simulink model "atrias_on_boom"  (R2018b)
settings: Solver=ode15s  StartTime=0.0  StopTime=inf  FixedStep=sample_time  MaxStep=1e-2  RelTol=1e-3
InitFcn:
  | addpath('../common/')
  | colors
  | simulation_params
  | mechanical_params
StartFcn:
  | clc
  | tic
StopFcn:
  | stopscript
values from neighbouring files (symbols this model uses):
  sample_time = 1/sample_freq    (= 0.001)    [simulation_params.m]
undefined symbols (not defined in the file or in its folder): Force_Control, rad, s, sgn, sm, t_friction, X, Y, Z
libraries: sm_lib x205, nesl_utility x123, simulink x49, fl_lib x16, mblibv1 x4, simulink_extras x2, powerlib_meascontrol x1
(part 5 of 8)

== system atrias_on_boom/Mechanical System Layer/R Leg/Thigh SEA ==
  note: Thigh SEA Mechanics
  Thigh Gear Torque [Nm] : Inport
  Thigh Joint [rad rad/s] : Inport  Port=2
  Continuous Angle : mblibv1/Utilities/Continuous Angle  rad=rad  rads=rad/s
      settings: SourceProductName=Simscape  SourceProductBaseCode=SS
  Demux : Demux  Outputs=2
  Gain : Gain  Gain=sm.k_leg_spring
  Gain1 : Gain  Gain=sm.b_leg_spring
  Initial Gear Angle : Constant  Value=sm.thigh_initial_r
  Inverse Gear Ratio1 : Gain  Gain=1/sm.N
  Inverse Gear Ratio2 : Gain  Gain=sm.Kt_leg
  Inverse Gear Ratio3 : Gain  Gain=1/sm.Kt_leg
  Motor Direction : Gain  Gain=-1
  Motor Efficiency : Gain  Gain=sm.mu_motor
  Motor Controller : Subsystem  Commented=on
  Motor Electromagnetism : Subsystem  Commented=on
  Rotor Damping : Gain  Gain=sm.b_rotor
  Rotor and Gearing : Subsystem
  Sum : Sum  Inputs=++|
  Sum2 : Sum  Inputs=+|-
  Sum3 : Sum  Inputs=|+-
  Sum4 : Sum  Inputs=+|-
  Sum5 : Sum  Inputs=|++
  Torque Limiter (outside) 2 : Saturate  UpperLimit=sm.LEG_MTR_MAX_TORQUE  LowerLimit=-sm.LEG_MTR_MAX_TORQUE  ZeroCross=off
      settings: AttributesFormatString=Hi: %<UpperLimit>\nLo: %<LowerLimit>
  Rotor Joint Conn : PMIOPort  Side=Left
  Thigh Joint Torque [Nm] : Outport
  Thigh Gear [rad] : Outport  Port=2
  wires:
  Sum2/1 -> Gain/1
  Sum3/1 -> Motor Efficiency/1
  Rotor Damping/1 -> Sum3/2
  Gain/1 -> Sum5/1  "tau_load"
  Gain1/1 -> Sum5/2
  Sum4/1 -> Gain1/1
  Thigh Joint [rad rad/s]/1 -> Demux/1
  Demux/1 -> Sum2/2
  Demux/2 -> Sum4/2
  Inverse Gear Ratio3/1 -> Inverse Gear Ratio2/1
  Inverse Gear Ratio2/1 -> Sum3/1
  Initial Gear Angle/1 -> Sum/1
  Sum/1 -> Thigh Gear [rad]/1, Sum2/1
  Continuous Angle/1 -> Sum/2
  Rotor and Gearing/1(Gearhead Position [rad]) -> Continuous Angle/1
  Motor Controller/1(Voltage [V]) -> Motor Electromagnetism/1(Voltage [V])
  Motor Electromagnetism/1(Current [A]) -> Motor Controller/2(Measured Current [A])
  Thigh Gear Torque [Nm]/1 -> Motor Direction/1
  Inverse Gear Ratio1/1 -> Inverse Gear Ratio3/1
  Motor Efficiency/1 -> Rotor and Gearing/1(Rotor Torque [Nm])
  Rotor and Gearing/2(Gearhead Velocity [rad/s]) -> Sum4/1, Continuous Angle/2
  Sum5/1 -> Thigh Joint Torque [Nm]/1, Rotor and Gearing/2(Spring Torque [Nm])
  Rotor and Gearing/3(Rotor Velocity [rad/s]) -> Rotor Damping/1
  Torque Limiter (outside) 2/1 -> Inverse Gear Ratio1/1
  Motor Direction/1 -> Torque Limiter (outside) 2/1
  connections:
  Rotor and Gearing/LConn1 -- Rotor Joint Conn/RConn1

== system atrias_on_boom/Mechanical System Layer/Right Hip Roll Joint/Mechanical Limits  ==
  vphi : Inport
  phi : Inport  Port=2
  Compare To Constant5 : simulink/Logic and Bit Operations/Compare To Constant  relop=<=  const=sm.phi_max_collision  OutDataTypeStr=boolean  ZeroCross=off
  Compare To Zero1 : simulink/Logic and Bit Operations/Compare To Zero  relop=<=  OutDataTypeStr=boolean  ZeroCross=off
  Compare To Zero2 : simulink/Logic and Bit Operations/Compare To Zero  relop=<=  OutDataTypeStr=boolean  ZeroCross=off
  Constant1 : Constant  Value=sm.phi_roll_min
  Constant2 : Constant  Value=sm.phi_roll_max
  Enabled Subsystem : Subsystem  TreatAsAtomicUnit=on
  Gain2 : Gain  Gain=-1
  Logical Operator : Logic  Operator=OR  Inputs=1  AllPortsSameDT=off  OutDataTypeStr=boolean
  Mux : Mux  Inputs=2
  Roll Max Collision Model : Subsystem
  Roll Min Collision Model : Subsystem
  Stop Simulation6 : Stop
  Sum1 : Sum  Inputs=-+|
  Sum11 : Sum  Inputs=-|+
  Sum5 : Sum  Inputs=+-|
  tau_reaction : Outport
  wires:
  Sum1/1 -> [col_hip_min], Compare To Zero1/1, Roll Min Collision Model/1(phi [rad])
  Roll Min Collision Model/1(tau_interaction[Nm]) -> Sum11/2
  Compare To Zero1/1 -> Roll Min Collision Model/Enable
  phi/1 -> Sum1/2, Sum5/2
  Logical Operator/1 -> Stop Simulation6/1, Enabled Subsystem/Enable
  [col_hip_max] -> Mux/1
  Mux/1 -> Compare To Constant5/1
  [col_hip_min] -> Mux/2
  Sum11/1 -> tau_reaction/1
  Constant1/1 -> Sum1/1
  Compare To Constant5/1 -> Enabled Subsystem/1(Col_Flags), Logical Operator/1
  Constant2/1 -> Sum5/1
  Sum5/1 -> [col_hip_max], Compare To Zero2/1, Roll Max Collision Model/1(phi [rad])
  Compare To Zero2/1 -> Roll Max Collision Model/Enable
  Roll Max Collision Model/1(tau_interaction[Nm]) -> Sum11/1
  vphi/1 -> Roll Min Collision Model/2(vphi [rad/s]), Gain2/1
  Gain2/1 -> Roll Max Collision Model/2(vphi [rad/s])

== system atrias_on_boom/Mechanical System Layer/Torso/Frame Data ==
  Kinematic Data : ToWorkspace  VariableName=torso_out  SampleTime=sm.output_sample_time
      settings: Save2DSignal=2-D array (concatenate along first dimension)
  Mux : Mux
  PS-Simulink Converter{,1..3} (4 alike) : nesl_utility/PS-Simulink Converter  PhysicalDomain=network_engine_domain  SubClassName=ps_output  LeftPortType=input  RightPortType=output  PseudoPeriodic=off  Frequencies=[]  Unit=1  AffineConversion=off
  Transform Sensor : sm_lib/Frames and Transforms/Transform Sensor  MeasurementFrame=World  SenseAngle=off  SenseAxis=off  SenseAngle1=off  SenseAngle2=off  SenseAngle3=off  SenseQ=on  SenseR=off  SenseOmegaX=off  SenseOmegaY=off  SenseOmegaZ=off  SenseOmega1=off  SenseOmega2=off  SenseOmega3=off  SenseQDot=off  SenseRDot=off  SenseAlphaX=off  SenseAlphaY=off  SenseAlphaZ=off  SenseAlpha1=off  SenseAlpha2=off  SenseAlpha3=off  SenseQDDot=off  SenseRDDot=off  SenseX=on  SenseY=on  SenseZ=on  SenseRad=off  SenseAzim=off  SenseDist=off  SenseInc=off  SenseXDot=off  SenseYDot=off  SenseZDot=off  SenseRadDot=off  SenseAzimDot=off  SenseDistDot=off  SenseIncDot=off  SenseXDDot=off  SenseYDDot=off  SenseZDDot=off  SenseRadDDot=off  SenseAzimDDot=off  SenseDistDDot=off  SenseIncDDot=off
  World Frame : sm_lib/Frames and Transforms/World Frame
  Frame : PMIOPort  Side=Left
  wires:
  Mux/1 -> Kinematic Data/1
  PS-Simulink Converter/1 -> Mux/1
  PS-Simulink Converter1/1 -> Mux/2
  PS-Simulink Converter2/1 -> Mux/3
  PS-Simulink Converter3/1 -> Mux/4
  connections:
  PS-Simulink Converter3/LConn1 -- Transform Sensor/RConn5
  PS-Simulink Converter2/LConn1 -- Transform Sensor/RConn4
  PS-Simulink Converter1/LConn1 -- Transform Sensor/RConn3
  PS-Simulink Converter/LConn1 -- Transform Sensor/RConn2
  Transform Sensor/RConn1 -- Frame/RConn1
  Transform Sensor/LConn1 -- World Frame/RConn1

== system atrias_on_boom/Mechanical System Layer/Yaw Shaft/Frame Data ==
  Kinematic Data : ToWorkspace  VariableName=boom_yaw_out  SampleTime=sm.output_sample_time
      settings: Save2DSignal=2-D array (concatenate along first dimension)
  Mux : Mux
  PS-Simulink Converter{,1..3} (4 alike) : nesl_utility/PS-Simulink Converter  PhysicalDomain=network_engine_domain  SubClassName=ps_output  LeftPortType=input  RightPortType=output  PseudoPeriodic=off  Frequencies=[]  Unit=1  AffineConversion=off
  Transform Sensor : sm_lib/Frames and Transforms/Transform Sensor  MeasurementFrame=World  SenseAngle=off  SenseAxis=off  SenseAngle1=off  SenseAngle2=off  SenseAngle3=off  SenseQ=on  SenseR=off  SenseOmegaX=off  SenseOmegaY=off  SenseOmegaZ=off  SenseOmega1=off  SenseOmega2=off  SenseOmega3=off  SenseQDot=off  SenseRDot=off  SenseAlphaX=off  SenseAlphaY=off  SenseAlphaZ=off  SenseAlpha1=off  SenseAlpha2=off  SenseAlpha3=off  SenseQDDot=off  SenseRDDot=off  SenseX=on  SenseY=on  SenseZ=on  SenseRad=off  SenseAzim=off  SenseDist=off  SenseInc=off  SenseXDot=off  SenseYDot=off  SenseZDot=off  SenseRadDot=off  SenseAzimDot=off  SenseDistDot=off  SenseIncDot=off  SenseXDDot=off  SenseYDDot=off  SenseZDDot=off  SenseRadDDot=off  SenseAzimDDot=off  SenseDistDDot=off  SenseIncDDot=off
  World Frame : sm_lib/Frames and Transforms/World Frame
  Frame : PMIOPort  Side=Left
  wires:
  Mux/1 -> Kinematic Data/1
  PS-Simulink Converter/1 -> Mux/1
  PS-Simulink Converter1/1 -> Mux/2
  PS-Simulink Converter2/1 -> Mux/3
  PS-Simulink Converter3/1 -> Mux/4
  connections:
  PS-Simulink Converter3/LConn1 -- Transform Sensor/RConn5
  PS-Simulink Converter2/LConn1 -- Transform Sensor/RConn4
  PS-Simulink Converter1/LConn1 -- Transform Sensor/RConn3
  PS-Simulink Converter/LConn1 -- Transform Sensor/RConn2
  Transform Sensor/RConn1 -- Frame/RConn1
  Transform Sensor/LConn1 -- World Frame/RConn1

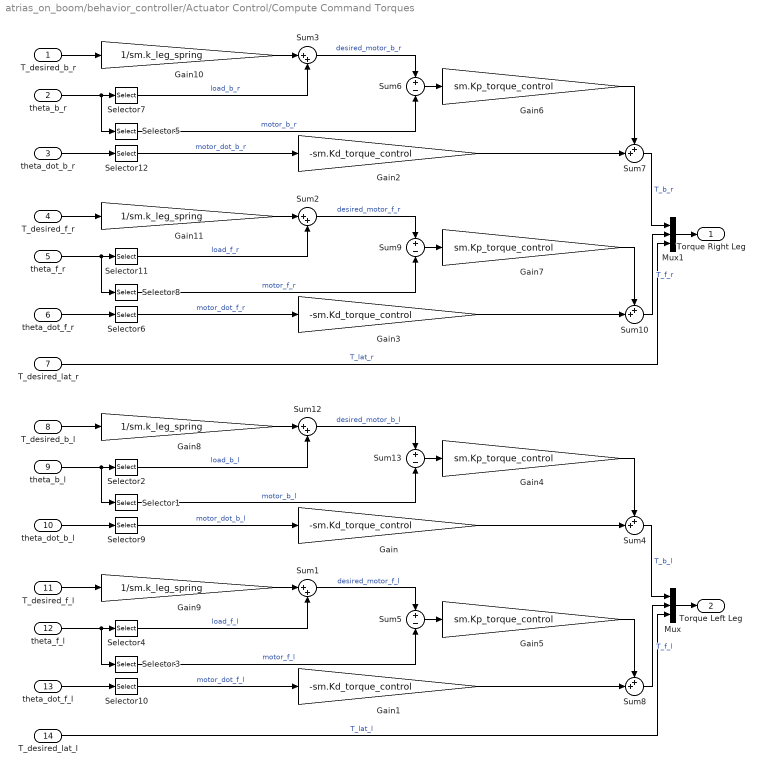
== system atrias_on_boom/behavior_controller/Actuator Control/Compute Command Torques ==
  T_desired_b_r : Inport
  theta_b_r : Inport  Port=2
  theta_dot_b_r : Inport  Port=3
  T_desired_f_r : Inport  Port=4
  theta_f_r : Inport  Port=5
  theta_dot_f_r : Inport  Port=6
  T_desired_lat_r : Inport  Port=7
  T_desired_b_l : Inport  Port=8
  theta_b_l : Inport  Port=9
  theta_dot_b_l : Inport  Port=10
  T_desired_f_l : Inport  Port=11
  theta_f_l : Inport  Port=12
  theta_dot_f_l : Inport  Port=13
  T_desired_lat_l : Inport  Port=14
  Gain{,1..3} (4 alike) : Gain  Gain=-sm.Kd_torque_control
  Gain{8..11} (4 alike) : Gain  Gain=1/sm.k_leg_spring
  Gain{4..7} (4 alike) : Gain  Gain=sm.Kp_torque_control
  Mux : Mux  Inputs=3
  Mux1 : Mux  Inputs=3
  Selector{1,3,5..6,8..10,12} (8 alike) : Selector  InputPortWidth=2  IndexOptions=Index vector (dialog)  Indices=[2]  OutputSizes=1
  Selector{2,4,7,11} (4 alike) : Selector  InputPortWidth=2  IndexOptions=Index vector (dialog)  Indices=[1]  OutputSizes=1
  Sum{1..3,12} (4 alike) : Sum  Inputs=|++
  Sum{4,7..8,10} (4 alike) : Sum  Inputs=++|
  Sum{5..6,9,13} (4 alike) : Sum  Inputs=+-
  Torque Right Leg : Outport
  Torque Left Leg : Outport  Port=2
  wires:
  Mux/1 -> Torque Left Leg/1
  Sum4/1 -> Mux/1  "T_b_l"
  Selector1/1 -> Sum13/2  "motor_b_l"
  Selector2/1 -> Sum12/2  "load_b_l"
  theta_b_l/1 -> Selector1/1, Selector2/1
  Selector9/1 -> Gain/1  "motor_dot_b_l"
  theta_dot_b_l/1 -> Selector9/1
  T_desired_b_l/1 -> Gain8/1
  Gain8/1 -> Sum12/1
  Sum12/1 -> Sum13/1  "desired_motor_b_l"
  Sum13/1 -> Gain4/1
  Gain/1 -> Sum4/2
  Gain4/1 -> Sum4/1
  Sum5/1 -> Gain5/1
  Selector4/1 -> Sum1/2  "load_f_l"
  Gain5/1 -> Sum8/1
  Selector10/1 -> Gain1/1  "motor_dot_f_l"
  theta_dot_f_l/1 -> Selector10/1
  Gain1/1 -> Sum8/2
  Gain9/1 -> Sum1/1
  Selector3/1 -> Sum5/2  "motor_f_l"
  Sum1/1 -> Sum5/1  "desired_motor_f_l"
  theta_f_l/1 -> Selector3/1, Selector4/1
  T_desired_f_l/1 -> Gain9/1
  Sum8/1 -> Mux/2  "T_f_l"
  T_desired_lat_l/1 -> Mux/3  "T_lat_l"
  Sum10/1 -> Mux1/2  "T_f_r"
  Selector11/1 -> Sum2/2  "load_f_r"
  Sum6/1 -> Gain6/1
  Sum7/1 -> Mux1/1  "T_b_r"
  Selector7/1 -> Sum3/2  "load_b_r"
  Gain7/1 -> Sum10/1
  Gain10/1 -> Sum3/1
  Sum2/1 -> Sum9/1  "desired_motor_f_r"
  theta_dot_f_r/1 -> Selector6/1
  theta_b_r/1 -> Selector5/1, Selector7/1
  T_desired_b_r/1 -> Gain10/1
  T_desired_lat_r/1 -> Mux1/3  "T_lat_r"
  Sum3/1 -> Sum6/1  "desired_motor_b_r"
  Selector6/1 -> Gain3/1  "motor_dot_f_r"
  Mux1/1 -> Torque Right Leg/1
  Gain2/1 -> Sum7/2
  Gain6/1 -> Sum7/1
  Selector12/1 -> Gain2/1  "motor_dot_b_r"
  Gain3/1 -> Sum10/2
  theta_dot_b_r/1 -> Selector12/1
  Selector5/1 -> Sum6/2  "motor_b_r"
  Gain11/1 -> Sum2/1
  T_desired_f_r/1 -> Gain11/1
  Selector8/1 -> Sum9/2  "motor_f_r"
  theta_f_r/1 -> Selector8/1, Selector11/1
  Sum9/1 -> Gain7/1

== system atrias_on_boom/behavior_controller/Behavior/Contact Detection ==
  Torque Left Leg : Inport
  theta_b_l : Inport  Port=2
  theta_f_l : Inport  Port=3
  Torque Right Leg : Inport  Port=4
  theta_b_r : Inport  Port=5
  theta_f_r : Inport  Port=6
  Demux : Demux  Outputs=2
  Demux2 : Demux  Outputs=2
  Divide : Product  Inputs=*/
  Divide1 : Product  Inputs=*/
  Dot Product : DotProduct  InputSameDT=on  OutDataTypeStr=Inherit: Inherit via internal rule
  Dot Product1 : DotProduct  InputSameDT=on  OutDataTypeStr=Inherit: Inherit via internal rule
  Gain : Gain  Gain=0.5
  Gain1 : Gain  Gain=0.5
  GreaterThan : RelationalOperator  Operator=<  OutDataTypeStr=boolean  RndMeth=Simplest
  GreaterThan1 : RelationalOperator  Operator=<  OutDataTypeStr=boolean  RndMeth=Simplest
  Half of total weight : Constant  Value=sm.g*sm.m_total*0.5
  NOT : Logic  Operator=NOT  IconShape=distinctive  AllPortsSameDT=off  OutDataTypeStr=boolean
  NOT1 : Logic  Operator=NOT  IconShape=distinctive  AllPortsSameDT=off  OutDataTypeStr=boolean
  Selector{,1..3} (4 alike) : Selector  InputPortWidth=2  IndexOptions=Index vector (dialog)  Indices=[1]  OutputSizes=1
  Sum : Sum  Inputs=+-
  Sum1 : Sum  Inputs=+-
  Sum2 : Sum  Inputs=-+
  Sum3 : Sum  Inputs=-+
  Trigonometric Function : Trigonometry
  Trigonometric Function1 : Trigonometry
  Left Leg in Swing? : Outport
  Both in Swing? : Outport  Port=2
  Both in Contact? : Outport  Port=3
  Right Leg in Swing? : Outport  Port=4
  wires:
  Torque Left Leg/1 -> Demux/1
  Demux/1 -> Sum/1
  Demux/2 -> Sum/2
  Torque Right Leg/1 -> Demux2/1
  Demux2/1 -> Sum1/1
  Demux2/2 -> Sum1/2
  Sum/1 -> Gain/1
  Sum1/1 -> Gain1/1
  theta_f_l/1 -> Selector1/1
  theta_b_l/1 -> Selector/1
  theta_f_r/1 -> Selector3/1
  theta_b_r/1 -> Selector2/1
  Sum3/1 -> Trigonometric Function/1
  Sum2/1 -> Trigonometric Function1/1
  Gain/1 -> Divide/1
  Trigonometric Function1/1 -> Divide/2
  Gain1/1 -> Divide1/1
  Trigonometric Function/1 -> Divide1/2
  Divide/1 -> GreaterThan/1  "F_leg_left"
  Divide1/1 -> GreaterThan1/1  "F_leg_right"
  Half of total weight/1 -> GreaterThan1/2, GreaterThan/2
  GreaterThan/1 -> Dot Product/1, NOT/1, Left Leg in Swing?/1
  GreaterThan1/1 -> NOT1/1, Dot Product/2, Right Leg in Swing?/1
  Dot Product/1 -> Both in Swing?/1
  Dot Product1/1 -> Both in Contact?/1
  NOT/1 -> Dot Product1/1
  NOT1/1 -> Dot Product1/2
  Selector/1 -> Sum2/1
  Selector1/1 -> Sum2/2
  Selector2/1 -> Sum3/1
  Selector3/1 -> Sum3/2

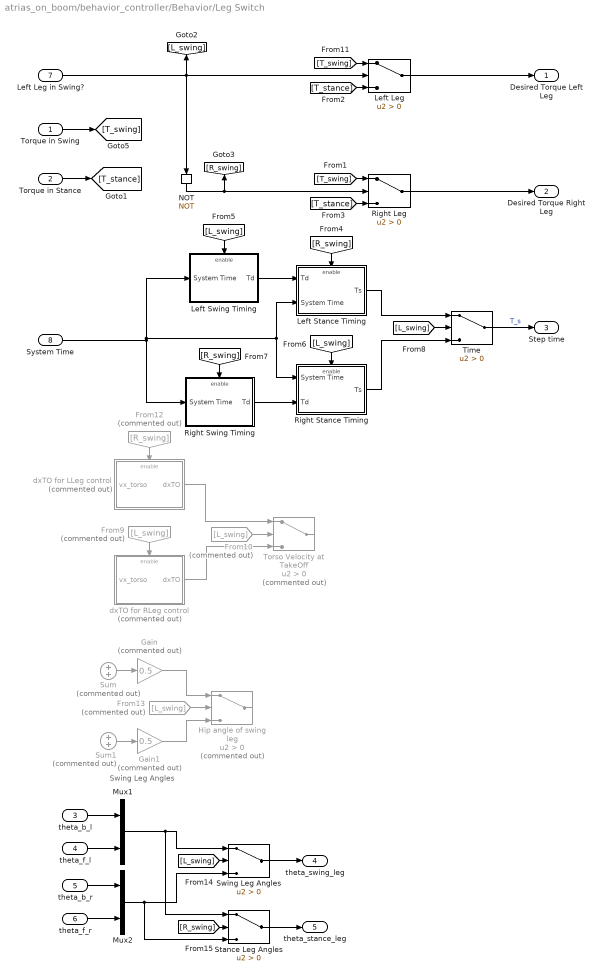
== system atrias_on_boom/behavior_controller/Behavior/Leg Switch ==
  note: Swing Leg Angles
  Torque in Swing : Inport
  Torque in Stance : Inport  Port=2
  theta_b_l : Inport  Port=3
  theta_f_l : Inport  Port=4
  theta_b_r : Inport  Port=5
  theta_f_r : Inport  Port=6
  "Left Leg in Swing? " : Inport  Port=7
  System Time : Inport  Port=8
  From10 : From  Commented=on  GotoTag=L_swing
  From12 : From  Commented=on  GotoTag=R_swing
  From13 : From  Commented=on  GotoTag=L_swing
  From9 : From  Commented=on  GotoTag=L_swing
  Gain : Gain  Commented=on  Gain=0.5
  Gain1 : Gain  Commented=on  Gain=0.5
  Hip angle of swing leg : Switch  Commented=on  Criteria=u2 > Threshold
  Left Leg : Switch  Criteria=u2 > Threshold
  Left Stance Timing : Subsystem
  Left Swing Timing : Subsystem
  Mux1 : Mux  Inputs=2
  Mux2 : Mux  Inputs=2
  NOT : Logic  Operator=NOT  IconShape=distinctive  AllPortsSameDT=off  OutDataTypeStr=boolean
  Right Leg : Switch  Criteria=u2 > Threshold
  Right Stance Timing : Subsystem
  Right Swing Timing : Subsystem
  Stance Leg Angles : Switch  Criteria=u2 > Threshold
  Sum : Sum  Commented=on
  Sum1 : Sum  Commented=on
  Swing Leg Angles : Switch  Criteria=u2 > Threshold
  Time : Switch  Criteria=u2 > Threshold
  Torso Velocity at TakeOff : Switch  Commented=on  Criteria=u2 > Threshold
  dxTO for LLeg control : Subsystem  Commented=on
  dxTO for RLeg control : Subsystem  Commented=on
  Desired Torque Left Leg : Outport
  Desired Torque Right Leg : Outport  Port=2
  Step time : Outport  Port=3
  theta_swing_leg : Outport  Port=4
  theta_stance_leg : Outport  Port=5
  wires:
  "Left Leg in Swing? "/1 -> NOT/1, Left Leg/2, [L_swing]
  NOT/1 -> [R_swing], Right Leg/2
  Torque in Swing/1 -> [T_swing]
  Torque in Stance/1 -> [T_stance]
  [T_swing] -> Left Leg/1
  [T_swing] -> Right Leg/1
  [T_stance] -> Left Leg/3
  [T_stance] -> Right Leg/3
  Left Leg/1 -> Desired Torque Left Leg/1
  Left Swing Timing/1(Td) -> Left Stance Timing/1(Td)
  Right Swing Timing/1(Td) -> Right Stance Timing/2(Td)
  [L_swing] -> Left Swing Timing/Enable
  [L_swing] -> Right Stance Timing/Enable
  [R_swing] -> Left Stance Timing/Enable
  [R_swing] -> Right Swing Timing/Enable
  Time/1 -> Step time/1  "T_s"
  Left Stance Timing/1(Ts) -> Time/1
  Right Stance Timing/1(Ts) -> Time/3
  [L_swing] -> Time/2
  From9/1 -> dxTO for RLeg control/Enable
  From12/1 -> dxTO for LLeg control/Enable
  dxTO for LLeg control/1(dxTO) -> Torso Velocity at TakeOff/1
  From10/1 -> Torso Velocity at TakeOff/2
  dxTO for RLeg control/1(dxTO) -> Torso Velocity at TakeOff/3
  Sum/1 -> Gain/1
  Sum1/1 -> Gain1/1
  From13/1 -> Hip angle of swing leg/2
  Gain/1 -> Hip angle of swing leg/1
  Gain1/1 -> Hip angle of swing leg/3
  theta_b_l/1 -> Mux1/1
  theta_f_l/1 -> Mux1/2
  theta_b_r/1 -> Mux2/1
  theta_f_r/1 -> Mux2/2
  [L_swing] -> Swing Leg Angles/2
  Swing Leg Angles/1 -> theta_swing_leg/1
  Stance Leg Angles/1 -> theta_stance_leg/1
  Mux2/1 -> Stance Leg Angles/3, Swing Leg Angles/3
  Mux1/1 -> Stance Leg Angles/1, Swing Leg Angles/1
  [R_swing] -> Stance Leg Angles/2
  Right Leg/1 -> Desired Torque Right Leg/1
  System Time/1 -> Left Swing Timing/1(System Time), Left Stance Timing/2(System Time), Right Stance Timing/1(System Time), Right Swing Timing/1(System Time)

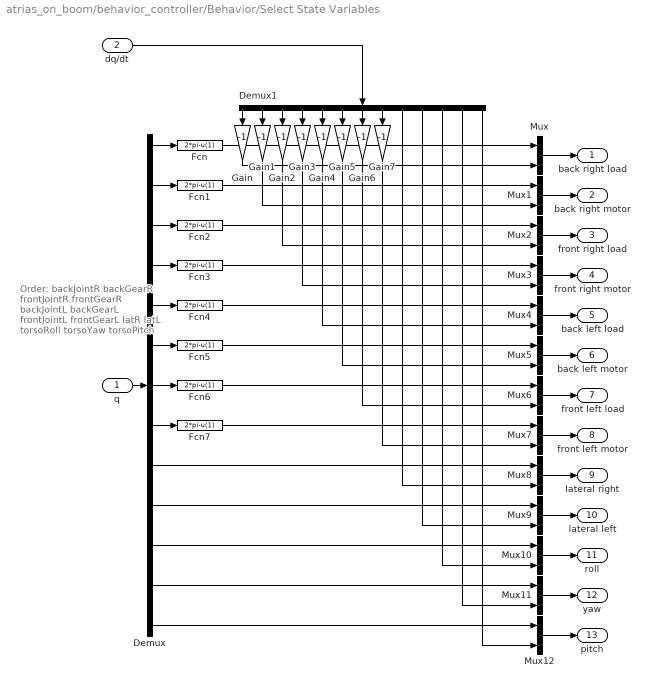
== system atrias_on_boom/behavior_controller/Behavior/Select State Variables ==
  note: Order:
      |
      | backJointR
      | backGearR
      | frontJointR
      | frontGearR
      |
      | backJointL
      | backGearL
      | frontJointL
      | frontGearL
      |
      | latR
      | latL
      |
      | torsoRoll
      | torsoYaw
      | torsoPitch
  q : Inport
  dq/dt : Inport  Port=2
  Demux : Demux  Outputs=13
  Demux1 : Demux  Outputs=13
  Fcn{,1..7} (8 alike) : Fcn  Expr=2*pi-u(1)
  Gain{,1..7} (8 alike) : Gain  Gain=-1
  Mux{,1..12} (13 alike) : Mux  Inputs=2
  back right load : Outport
  back right motor : Outport  Port=2
  front right load : Outport  Port=3
  front right motor : Outport  Port=4
  back left load : Outport  Port=5
  back left motor : Outport  Port=6
  front left load : Outport  Port=7
  front left motor : Outport  Port=8
  lateral right : Outport  Port=9
  lateral left : Outport  Port=10
  roll : Outport  Port=11
  yaw : Outport  Port=12
  pitch : Outport  Port=13
  wires:
  q/1 -> Demux/1
  Mux/1 -> back right load/1
  Mux1/1 -> back right motor/1
  Mux4/1 -> back left load/1
  Mux5/1 -> back left motor/1
  Mux8/1 -> lateral right/1
  Mux9/1 -> lateral left/1
  Mux12/1 -> pitch/1
  Mux2/1 -> front right load/1
  Mux3/1 -> front right motor/1
  Mux6/1 -> front left load/1
  Mux7/1 -> front left motor/1
  Mux10/1 -> roll/1
  Mux11/1 -> yaw/1
  Demux/1 -> Fcn/1
  Demux1/1 -> Gain/1
  Demux/2 -> Fcn1/1
  Demux/3 -> Fcn2/1
  Demux/4 -> Fcn3/1
  Demux/5 -> Fcn4/1
  Demux/6 -> Fcn5/1
  Demux/7 -> Fcn6/1
  Demux/8 -> Fcn7/1
  Demux/10 -> Mux9/1
  Demux/11 -> Mux10/1
  Demux/12 -> Mux11/1
  Demux/13 -> Mux12/1
  Demux1/2 -> Gain1/1
  Demux1/3 -> Gain2/1
  Demux1/4 -> Gain3/1
  Demux1/5 -> Gain4/1
  Demux1/6 -> Gain5/1
  Demux1/7 -> Gain6/1
  Demux1/8 -> Gain7/1
  Demux1/9 -> Mux8/2
  Demux1/10 -> Mux9/2
  Demux1/11 -> Mux10/2
  Demux1/12 -> Mux11/2
  Demux1/13 -> Mux12/2
  dq/dt/1 -> Demux1/1
  Fcn/1 -> Mux/1
  Fcn1/1 -> Mux1/1
  Fcn2/1 -> Mux2/1
  Fcn3/1 -> Mux3/1
  Fcn4/1 -> Mux4/1
  Fcn5/1 -> Mux5/1
  Fcn6/1 -> Mux6/1
  Fcn7/1 -> Mux7/1
  Demux/9 -> Mux8/1
  Gain/1 -> Mux/2
  Gain1/1 -> Mux1/2
  Gain2/1 -> Mux2/2
  Gain3/1 -> Mux3/2
  Gain4/1 -> Mux4/2
  Gain5/1 -> Mux5/2
  Gain6/1 -> Mux6/2
  Gain7/1 -> Mux7/2

== system atrias_on_boom/behavior_controller/Behavior/Stance Leg Control ==
  note: Simplified Inverse Dynamics Model
      | LegForces -> Joint Torques
  Torso Pitch : Inport
  Stance Leg Angle : Inport  Port=2
  vx_torso : Inport  Port=3
  vz_torso : Inport  Port=4
  z_torso : Inport  Port=5
  "torso_roll " : Inport  Port=6
  Constant : Constant  Value=sm.F_thrust
  Demux : Demux  Outputs=2
  Gain : Gain  Gain=sm.l_seg
  Gain1 : Gain  Gain=sm.Kp_lateral
  Gain2 : Gain  Gain=sm.Kd_lateral
  Mux : Mux  Inputs=3
  Mux1 : Mux  Inputs=3
  Product : Product
  Selector : Selector  InputPortWidth=4  IndexOptions=Index vector (dialog)  Indices=[1 3]  OutputSizes=1
  Selector1 : Selector  InputPortWidth=2  IndexOptions=Index vector (dialog)  Indices=[1]  OutputSizes=1
  Selector2 : Selector  InputPortWidth=2  IndexOptions=Index vector (dialog)  Indices=[2]  OutputSizes=1
  Sum : Sum  Inputs=-+
  Sum1 : Sum  Inputs=|++
  Sum2 : Sum  Inputs=|+-
  Sum3 : Sum  Inputs=|++
  Sum4 : Sum  Inputs=|++
  Torque for centripetal force : Fcn  Expr=sm.m_total*(u(1)^2+u(2)^2)/sm.l_boom*u(3)
  Trigonometric Function : Trigonometry
  Trunk Pitch Control : Fcn  Expr=sm.Kp_hip*(0-u(1)) + sm.Kd_hip*(0-u(2))
  Desired Stance Torques : Outport  OutputWhenDisabled=reset  InitialOutput=0
  wires:
  Torso Pitch/1 -> Trunk Pitch Control/1
  Trunk Pitch Control/1 -> Sum2/1, Sum1/1  "Leg torque"
  Mux/1 -> Desired Stance Torques/1
  Constant/1 -> Product/1  "Leg force"
  Stance Leg Angle/1 -> Selector/1
  Demux/1 -> Sum/1  "b"
  Demux/2 -> Sum/2  "f"
  Sum/1 -> Trigonometric Function/1
  Trigonometric Function/1 -> Gain/1
  Gain/1 -> Product/2
  Product/1 -> Sum1/2, Sum2/2
  Sum2/1 -> Mux/2  "T_f"
  Sum1/1 -> Mux/1  "T_b"
  Selector/1 -> Demux/1
  vz_torso/1 -> Mux1/2
  vx_torso/1 -> Mux1/1
  z_torso/1 -> Mux1/3
  Mux1/1 -> Torque for centripetal force/1
  Torque for centripetal force/1 -> Sum4/1  "T_centripetal"
  "torso_roll "/1 -> Selector2/1, Selector1/1
  Gain2/1 -> Sum3/1
  Gain1/1 -> Sum3/2
  Sum3/1 -> Sum4/2  "T_tipping"
  Sum4/1 -> Mux/3  "T_lat"
  Selector1/1 -> Gain1/1
  Selector2/1 -> Gain2/1

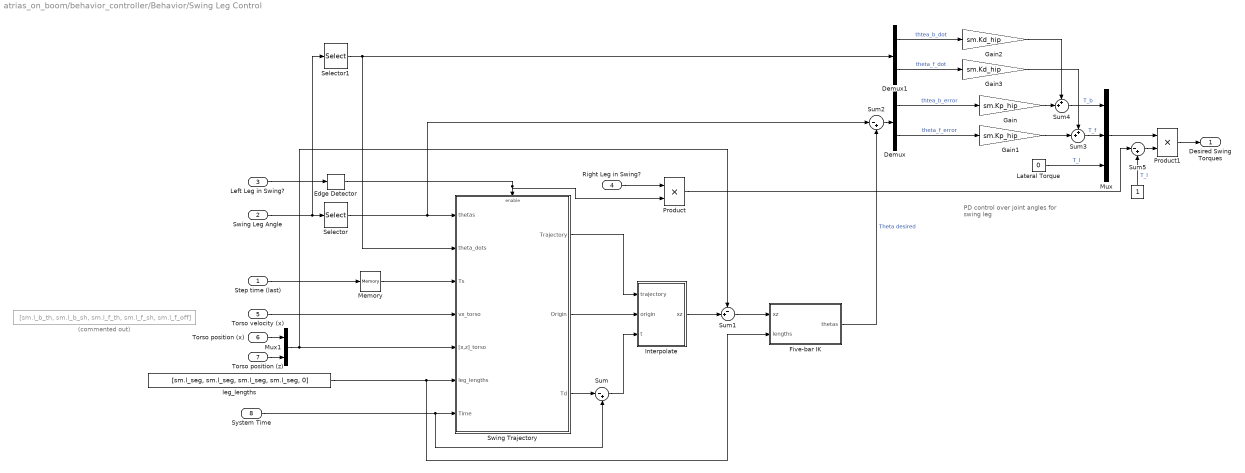
== system atrias_on_boom/behavior_controller/Behavior/Swing Leg Control ==
  note: PD control over joint angles
      | for swing leg
  Step time (last) : Inport
  Swing Leg Angle : Inport  Port=2
  Left Leg in Swing? : Inport  Port=3
  Right Leg in Swing? : Inport  Port=4
  Torso velocity (x) : Inport  Port=5
  Torso position (x) : Inport  Port=6
  Torso position (z) : Inport  Port=7
  System Time : Inport  Port=8
  " " : Constant  Commented=on  Value=[sm.l_b_th, sm.l_b_sh, sm.l_f_th, sm.l_f_sh, sm.l_f_off]
  "  " : Constant
  " Lateral Torque" : Constant  Value=0
  Demux : Demux  Outputs=2
  Demux1 : Demux  Outputs=2
  Edge Detector : powerlib_meascontrol/Logic/Edge Detector  model=Either  ic=0  Ts=0
      settings: SourceProductName=Simscape Power Systems  SourceProductBaseCode=PS
  Five-bar IK : MATLAB Function  TreatAsAtomicUnit=on
  Gain : Gain  Gain=sm.Kp_hip
  Gain1 : Gain  Gain=sm.Kp_hip
  Gain2 : Gain  Gain=sm.Kd_hip
  Gain3 : Gain  Gain=sm.Kd_hip
  Interpolate : MATLAB Function  TreatAsAtomicUnit=on  SystemSampleTime=0.005
  Memory : Memory  InitialCondition=sm.Ts
  Mux : Mux  Inputs=3
  Mux1 : Mux  Inputs=2
  Product : Product
  Product1 : Product
  Selector : Selector  InputPortWidth=4  IndexOptions=Index vector (dialog)  Indices=[1 3]  OutputSizes=1
  Selector1 : Selector  InputPortWidth=4  IndexOptions=Index vector (dialog)  Indices=[2 4]  OutputSizes=1
  Sum : Sum  Inputs=|-+
  Sum1 : Sum  Inputs=-+|
  Sum2 : Sum  Inputs=|-+
  Sum3 : Sum  Inputs=++|
  Sum4 : Sum  Inputs=++|
  Sum5 : Sum  Inputs=|-+
  Swing Trajectory : Subsystem
  leg_lengths : Constant  Value=[sm.l_seg, sm.l_seg, sm.l_seg, sm.l_seg, 0]
  Desired Swing Torques : Outport  OutputWhenDisabled=reset  InitialOutput=0
  wires:
  Left Leg in Swing?/1 -> Edge Detector/1
  Step time (last)/1 -> Memory/1
  Torso velocity (x)/1 -> Swing Trajectory/4(vx_torso)
  Torso position (x)/1 -> Mux1/1
  Torso position (z)/1 -> Mux1/2
  Mux1/1 -> Sum1/1, Swing Trajectory/5("[x,z]_torso")
  Swing Leg Angle/1 -> Selector1/1, Selector/1
  System Time/1 -> Swing Trajectory/7(Time), Sum/2
  Swing Trajectory/1(Trajectory) -> Interpolate/1(trajectory)
  Swing Trajectory/3(Td) -> Sum/1
  Sum/1 -> Interpolate/3(t)
  Swing Trajectory/2(Origin) -> Interpolate/2(origin)
  leg_lengths/1 -> Swing Trajectory/6(leg_lengths), Five-bar IK/2(lengths)
  Interpolate/1(xz) -> Sum1/2
  Sum1/1 -> Five-bar IK/1(xz)
  Five-bar IK/1(thetas) -> Sum2/2  "Theta desired"
  Demux/1 -> Gain/1  "thtea_b_error"
  Sum2/1 -> Demux/1
  Demux/2 -> Gain1/1  "theta_f_error"
  Gain/1 -> Sum4/2
  Gain2/1 -> Sum4/1
  Sum4/1 -> Mux/1  "T_b"
  Sum3/1 -> Mux/2  "T_f"
  Mux/1 -> Product1/1
  Memory/1 -> Swing Trajectory/3(Ts)
  Selector/1 -> Sum2/1, Swing Trajectory/1(thetas)
  Selector1/1 -> Swing Trajectory/2(theta_dots), Demux1/1
  Demux1/1 -> Gain2/1  "thtea_b_dot"
  Gain1/1 -> Sum3/2
  Demux1/2 -> Gain3/1  "theta_f_dot"
  Gain3/1 -> Sum3/1
  " Lateral Torque"/1 -> Mux/3  "T_l"
  Edge Detector/1 -> Swing Trajectory/Enable, Product/2
  Right Leg in Swing?/1 -> Product/1
  Product1/1 -> Desired Swing Torques/1
  "  "/1 -> Sum5/2  "T_l"
  Sum5/1 -> Product1/2
  Product/1 -> Sum5/1

== system atrias_on_boom/behavior_controller/Behavior/Torque ==
  theta_load_b_l : Inport
  theta_motor_b_l : Inport  Port=2
  theta_load_f_l : Inport  Port=3
  theta_motor_f_l : Inport  Port=4
  theta_load_b_r : Inport  Port=5
  theta_motor_b_r : Inport  Port=6
  theta_load_f_r : Inport  Port=7
  theta_motor_f_r : Inport  Port=8
  Gain{,1..3} (4 alike) : Gain  Gain=sm.k_leg_spring
  Gain{4..7} (4 alike) : Gain  Gain=sm.b_leg_spring
  Mux : Mux  Inputs=2
  Mux1 : Mux  Inputs=2
  Selector{1,3,5,7} (4 alike) : Selector  InputPortWidth=2  IndexOptions=Index vector (dialog)  Indices=[2]  OutputSizes=1
  Selector{2,4,6,8} (4 alike) : Selector  InputPortWidth=2  IndexOptions=Index vector (dialog)  Indices=[1]  OutputSizes=1
  Sum{,1..3} (4 alike) : Sum  Inputs=-+
  Sum{4..7} (4 alike) : Sum  Inputs=|++
  Torque Left Leg : Outport
  Torque Right Leg : Outport  Port=2
  wires:
  theta_motor_b_l/1 -> Sum/2
  theta_load_b_l/1 -> Sum/1
  Gain/1 -> Sum4/2
  Gain1/1 -> Sum5/2
  theta_motor_f_l/1 -> Sum1/2
  theta_load_f_l/1 -> Sum1/1
  Mux/1 -> Torque Left Leg/1
  theta_load_b_r/1 -> Sum2/1
  theta_motor_b_r/1 -> Sum2/2
  Mux1/1 -> Torque Right Leg/1
  theta_load_f_r/1 -> Sum3/1
  theta_motor_f_r/1 -> Sum3/2
  Gain4/1 -> Sum4/1
  Sum4/1 -> Mux/1  "T_b_l"
  Gain5/1 -> Sum5/1
  Sum5/1 -> Mux/2  "T_f_l"
  Gain2/1 -> Sum6/2
  Gain6/1 -> Sum6/1
  Sum6/1 -> Mux1/1  "T_b_r"
  Gain3/1 -> Sum7/2
  Gain7/1 -> Sum7/1
  Sum7/1 -> Mux1/2  "T_f_r"
  Sum/1 -> Selector1/1, Selector2/1
  Selector2/1 -> Gain/1
  Selector1/1 -> Gain4/1
  Sum1/1 -> Selector4/1, Selector3/1
  Selector4/1 -> Gain1/1
  Selector3/1 -> Gain5/1
  Sum2/1 -> Selector6/1, Selector5/1
  Selector5/1 -> Gain6/1
  Selector6/1 -> Gain2/1
  Sum3/1 -> Selector7/1, Selector8/1
  Selector7/1 -> Gain7/1
  Selector8/1 -> Gain3/1

== system atrias_on_boom/behavior_controller/Behavior/Torso ==
  note: Things to do:
      | Add filtering?
  Acceleration : Inport
  "Integrator, Second-Order" : SecondOrderIntegrator  ICX=0
  "Integrator, Second-Order1" : SecondOrderIntegrator  ICX=sm.initial_com_height
  x : Selector  InputPortWidth=3  IndexOptions=Index vector (dialog)  Indices=[1]  OutputSizes=1
  z : Selector  InputPortWidth=3  IndexOptions=Index vector (dialog)  Indices=[3]  OutputSizes=1
  vx_torso : Outport
  x_torso : Outport  Port=2
  vz_torso : Outport  Port=3
  z_torso : Outport  Port=4
  wires:
  Acceleration/1 -> z/1, x/1
  x/1 -> "Integrator, Second-Order"/1
  z/1 -> "Integrator, Second-Order1"/1
  "Integrator, Second-Order1"/2 -> vz_torso/1
  "Integrator, Second-Order"/2 -> vx_torso/1
  "Integrator, Second-Order"/1 -> x_torso/1
  "Integrator, Second-Order1"/1 -> z_torso/1

== system atrias_on_boom/Mechanical System Layer/L Ground Contact/Ground Friction Model/Friction Switch ==
  note: Static/Kinetic Friction Switch
  Slide! : Inport
  Stick! : Inport  Port=2
  Memory : Memory  InheritSampleTime=on
  S-R Flip-Flop : simulink_extras/Flip Flops/S-R Flip-Flop  initial_condition=0
  Terminator : Terminator
  Stiction : Outport
  wires:
  Memory/1 -> Stiction/1
  Slide!/1 -> S-R Flip-Flop/2
  Stick!/1 -> S-R Flip-Flop/1
  S-R Flip-Flop/2 -> Terminator/1
  S-R Flip-Flop/1 -> Memory/1

== system atrias_on_boom/Mechanical System Layer/L Ground Contact/Ground Friction Model/t-Axis Kinetic Friction Model ==
  note: Sliding Limit Detector
  note: Footpoint Determiner
  note: Kinetic Friction Model
  pos_x [m] : Inport
  vel_x [m/s] : Inport  Port=2
  pos_z [m] : Inport  Port=3
  vel_z [m/s] : Inport  Port=4
  F_Normal [N] : Inport  Port=5
  Enable : EnablePort  StatesWhenEnabling=reset  ZeroCross=off
  Constant : Constant  Value=sm.vLimit
  Constant1 : Constant  Value=eps
  Demux : Demux  Outputs=2
  Divide : Product  Inputs=*/
  FixPt Relational Operator : RelationalOperator  Operator=>  OutDataTypeStr=boolean  ZeroCross=off  RndMeth=Nearest
  Magnitude : Subsystem
  Memory : Memory  InheritSampleTime=on
  Mux : Mux  Inputs=2
  Negative : simulink/Logic and Bit Operations/Compare To Zero  relop=<  OutDataTypeStr=boolean
  Product : Product  RndMeth=Zero
  Sum : Sum  Inputs=|+-
  Sum1 : Sum  Inputs=|++
  reverse : Gain  Gain=-1
  sliding friction coefficient : Gain  Gain=sm.mu_slide
  posFP_x [m] : Outport  InitialOutput=0
      settings: AttributesFormatString=initial = '%<InitialOutput>'\nwhen disabled = '%<OutputWhenDisabled>'
  posFP_z [m] : Outport  Port=2  InitialOutput=0
      settings: AttributesFormatString=initial = '%<InitialOutput>'\nwhen disabled = '%<OutputWhenDisabled>'
  Stiction! : Outport  Port=3  OutputWhenDisabled=reset  InitialOutput=0
      settings: AttributesFormatString=initial = '%<InitialOutput>'\nwhen disabled = '%<OutputWhenDisabled>'
  Fx_Slide [N] : Outport  Port=4  OutputWhenDisabled=reset  InitialOutput=0
      settings: AttributesFormatString=initial = '%<InitialOutput>'\nwhen disabled = '%<OutputWhenDisabled>'
  Fz_Slide [N] : Outport  Port=5  OutputWhenDisabled=reset  InitialOutput=0
      settings: AttributesFormatString=initial = '%<InitialOutput>'\nwhen disabled = '%<OutputWhenDisabled>'
  wires:
  Demux/2 -> Fz_Slide [N]/1
  Demux/1 -> Fx_Slide [N]/1
  Product/1 -> Demux/1
  Sum1/1 -> Divide/2
  Constant1/1 -> Sum1/2
  Mux/1 -> Magnitude/1(Vector), Divide/1
  vel_z [m/s]/1 -> Mux/2
  vel_x [m/s]/1 -> Mux/1
  pos_z [m]/1 -> posFP_z [m]/1
  Constant/1 -> Sum/2
  Sum/1 -> Negative/1
  Magnitude/1(Magnitude) -> Sum1/1, Sum/1
  Negative/1 -> FixPt Relational Operator/1, Memory/1
  Memory/1 -> FixPt Relational Operator/2
  FixPt Relational Operator/1 -> Stiction!/1
  Divide/1 -> reverse/1
  sliding friction coefficient/1 -> Product/2
  pos_x [m]/1 -> posFP_x [m]/1
  F_Normal [N]/1 -> sliding friction coefficient/1
  reverse/1 -> Product/1

== system atrias_on_boom/Mechanical System Layer/L Ground Contact/Ground Friction Model/t-Axis Static Friction Model ==
  note: Static Friction Model
  note: Stiction Limit Detector
  note: Zero multiplication prevents
      | horizontal friction model from
      | oscillating between static and kinetic
      | friction when the vertical force is zero but
      | the ground level is not yet reached
      | in the upward motion
  F_Normal [N] : Inport
  pos_x [m] : Inport  Port=2
  vel_x [m/s] : Inport  Port=3
  pos_z [m] : Inport  Port=4
  vel_z [m/s] : Inport  Port=5
  posFP_x [m] : Inport  Port=6
  posFP_z [m] : Inport  Port=7
  Enable : EnablePort  StatesWhenEnabling=reset  ZeroCross=off
  Abs : Abs
  Check Vertical Friction : Product  RndMeth=Zero
  Check Vertical Friction1 : Product  RndMeth=Zero
  FixPt Relational Operator : RelationalOperator  Operator=>  OutDataTypeStr=boolean  ZeroCross=off  RndMeth=Nearest
  Gain1 : Gain  Gain=sm.k_gx
  Gain2 : Gain  Gain=1/sm.v_gx_max
  Gain3 : Gain  Gain=sm.k_gx
  Gain4 : Gain  Gain=1/sm.v_gx_max
  Magnitude : Subsystem
  Memory : Memory  InheritSampleTime=on
  Mux : Mux  Inputs=2
  Mux1 : Mux  Inputs=2
  Mux2 : Mux  Inputs=2
  Positive : simulink/Logic and Bit Operations/Compare To Zero  relop=>  OutDataTypeStr=boolean
  Positive1 : simulink/Logic and Bit Operations/Compare To Zero  relop=>  OutDataTypeStr=boolean
  Positive2 : simulink/Logic and Bit Operations/Compare To Zero  relop=>  OutDataTypeStr=boolean
  Sum : Sum  Inputs=-+
  Sum1 : Sum  Inputs=-+|
  Sum2 : Sum  Inputs=-+|
  X-Axis Stiction Force : Fcn  Expr=-u(1) * (1+sgn(u(1))*u(2))
  Z-Axis Stiction Force : Fcn  Expr=-u(1) * (1+sgn(u(1))*u(2))
  stiction limit force : Gain  Gain=sm.mu_stick
  Fz_Stick [N] : Outport  OutputWhenDisabled=reset  InitialOutput=0
      settings: AttributesFormatString=when disabled: %<OutputWhenDisabled>\ninitial: %<InitialOutput>
  Fx_Stick [N] : Outport  Port=2  OutputWhenDisabled=reset  InitialOutput=0
      settings: AttributesFormatString=when disabled: %<OutputWhenDisabled>\ninitial: %<InitialOutput>
  Sliding! : Outport  Port=3  OutputWhenDisabled=reset  InitialOutput=0
      settings: AttributesFormatString=when disabled: %<OutputWhenDisabled>\ninitial: %<InitialOutput>
  wires:
  Sum1/1 -> Gain1/1
  Mux/1 -> Magnitude/1(Vector)
  Magnitude/1(Magnitude) -> Sum/2
  Check Vertical Friction1/1 -> Fz_Stick [N]/1, Mux/1
  Z-Axis Stiction Force/1 -> Check Vertical Friction1/1
  Positive2/1 -> Check Vertical Friction1/2
  pos_z [m]/1 -> Sum1/2
  posFP_z [m]/1 -> Sum1/1
  vel_z [m/s]/1 -> Gain2/1
  Mux2/1 -> Z-Axis Stiction Force/1
  Gain1/1 -> Mux2/1
  Gain2/1 -> Mux2/2
  F_Normal [N]/1 -> stiction limit force/1, Positive1/1, Positive2/1
  Sum2/1 -> Gain3/1  "dx"
  pos_x [m]/1 -> Sum2/2
  posFP_x [m]/1 -> Sum2/1
  vel_x [m/s]/1 -> Gain4/1
  Sum/1 -> Positive/1
  Memory/1 -> FixPt Relational Operator/2
  Positive/1 -> FixPt Relational Operator/1, Memory/1
  Mux1/1 -> X-Axis Stiction Force/1
  Gain3/1 -> Mux1/1
  Gain4/1 -> Mux1/2
  FixPt Relational Operator/1 -> Sliding!/1
  Abs/1 -> Sum/1
  stiction limit force/1 -> Abs/1
  X-Axis Stiction Force/1 -> Check Vertical Friction/1
  Positive1/1 -> Check Vertical Friction/2
  Check Vertical Friction/1 -> Fx_Stick [N]/1, Mux/2

== system atrias_on_boom/Mechanical System Layer/L Leg/Four Bar Link/Frame Data ==
  Kinematic Data : ToWorkspace  VariableName=l_fb_link_out  SampleTime=sm.output_sample_time
      settings: Save2DSignal=2-D array (concatenate along first dimension)
  Mux : Mux
  PS-Simulink Converter{,1..3} (4 alike) : nesl_utility/PS-Simulink Converter  PhysicalDomain=network_engine_domain  SubClassName=ps_output  LeftPortType=input  RightPortType=output  PseudoPeriodic=off  Frequencies=[]  Unit=1  AffineConversion=off
  Transform Sensor : sm_lib/Frames and Transforms/Transform Sensor  MeasurementFrame=World  SenseAngle=off  SenseAxis=off  SenseAngle1=off  SenseAngle2=off  SenseAngle3=off  SenseQ=on  SenseR=off  SenseOmegaX=off  SenseOmegaY=off  SenseOmegaZ=off  SenseOmega1=off  SenseOmega2=off  SenseOmega3=off  SenseQDot=off  SenseRDot=off  SenseAlphaX=off  SenseAlphaY=off  SenseAlphaZ=off  SenseAlpha1=off  SenseAlpha2=off  SenseAlpha3=off  SenseQDDot=off  SenseRDDot=off  SenseX=on  SenseY=on  SenseZ=on  SenseRad=off  SenseAzim=off  SenseDist=off  SenseInc=off  SenseXDot=off  SenseYDot=off  SenseZDot=off  SenseRadDot=off  SenseAzimDot=off  SenseDistDot=off  SenseIncDot=off  SenseXDDot=off  SenseYDDot=off  SenseZDDot=off  SenseRadDDot=off  SenseAzimDDot=off  SenseDistDDot=off  SenseIncDDot=off
  World Frame : sm_lib/Frames and Transforms/World Frame
  Frame : PMIOPort  Side=Left
  wires:
  PS-Simulink Converter3/1 -> Mux/4
  PS-Simulink Converter2/1 -> Mux/3
  PS-Simulink Converter1/1 -> Mux/2
  PS-Simulink Converter/1 -> Mux/1
  Mux/1 -> Kinematic Data/1
  connections:
  Transform Sensor/LConn1 -- World Frame/RConn1
  Transform Sensor/RConn1 -- Frame/RConn1
  PS-Simulink Converter/LConn1 -- Transform Sensor/RConn2
  PS-Simulink Converter1/LConn1 -- Transform Sensor/RConn3
  PS-Simulink Converter2/LConn1 -- Transform Sensor/RConn4
  PS-Simulink Converter3/LConn1 -- Transform Sensor/RConn5

== system atrias_on_boom/Mechanical System Layer/L Leg/Lower Leg/Frame Data ==
  Kinematic Data : ToWorkspace  VariableName=l_lower_leg_out  SampleTime=sm.output_sample_time
      settings: Save2DSignal=2-D array (concatenate along first dimension)
  Mux : Mux
  PS-Simulink Converter{,1..3} (4 alike) : nesl_utility/PS-Simulink Converter  PhysicalDomain=network_engine_domain  SubClassName=ps_output  LeftPortType=input  RightPortType=output  PseudoPeriodic=off  Frequencies=[]  Unit=1  AffineConversion=off
  Transform Sensor : sm_lib/Frames and Transforms/Transform Sensor  MeasurementFrame=World  SenseAngle=off  SenseAxis=off  SenseAngle1=off  SenseAngle2=off  SenseAngle3=off  SenseQ=on  SenseR=off  SenseOmegaX=off  SenseOmegaY=off  SenseOmegaZ=off  SenseOmega1=off  SenseOmega2=off  SenseOmega3=off  SenseQDot=off  SenseRDot=off  SenseAlphaX=off  SenseAlphaY=off  SenseAlphaZ=off  SenseAlpha1=off  SenseAlpha2=off  SenseAlpha3=off  SenseQDDot=off  SenseRDDot=off  SenseX=on  SenseY=on  SenseZ=on  SenseRad=off  SenseAzim=off  SenseDist=off  SenseInc=off  SenseXDot=off  SenseYDot=off  SenseZDot=off  SenseRadDot=off  SenseAzimDot=off  SenseDistDot=off  SenseIncDot=off  SenseXDDot=off  SenseYDDot=off  SenseZDDot=off  SenseRadDDot=off  SenseAzimDDot=off  SenseDistDDot=off  SenseIncDDot=off
  World Frame : sm_lib/Frames and Transforms/World Frame
  Frame : PMIOPort  Side=Left
  wires:
  PS-Simulink Converter3/1 -> Mux/4
  PS-Simulink Converter2/1 -> Mux/3
  PS-Simulink Converter1/1 -> Mux/2
  PS-Simulink Converter/1 -> Mux/1
  Mux/1 -> Kinematic Data/1
  connections:
  Transform Sensor/LConn1 -- World Frame/RConn1
  Transform Sensor/RConn1 -- Frame/RConn1
  PS-Simulink Converter/LConn1 -- Transform Sensor/RConn2
  PS-Simulink Converter1/LConn1 -- Transform Sensor/RConn3
  PS-Simulink Converter2/LConn1 -- Transform Sensor/RConn4
  PS-Simulink Converter3/LConn1 -- Transform Sensor/RConn5

== system atrias_on_boom/Mechanical System Layer/L Leg/Mechanical Limits/Enabled Subsystem ==
  Col_Flags : Inport
  Enable : EnablePort  StatesWhenEnabling=reset  ZeroCross=off
  To Workspace : ToWorkspace  VariableName=L_collision_flags  SampleTime=-1
  wires:
  Col_Flags/1 -> To Workspace/1

== system atrias_on_boom/Mechanical System Layer/L Leg/Mechanical Limits/Shin Max Collision Model ==
  note: Mechanical Limits Model
  phi [rad] : Inport
  vphi [rad/s] : Inport  Port=2
  Contact! : EnablePort  StatesWhenEnabling=reset
  Gain3 : Gain  Gain=sm.k_phi
  Gain4 : Gain  Gain=1/sm.v_phi_max
  Mux1 : Mux  Inputs=2
  Reaction Force : Fcn  Expr="- u(1)  *  (1-u(2)) * (u(2)<1)"
  tau_interaction[Nm] : Outport  OutputWhenDisabled=reset  InitialOutput=0
      settings: AttributesFormatString=initial = '%<InitialOutput>'\nwhen disabled = '%<OutputWhenDisabled>'
  wires:
  Reaction Force/1 -> tau_interaction[Nm]/1
  phi [rad]/1 -> Gain3/1
  vphi [rad/s]/1 -> Gain4/1
  Mux1/1 -> Reaction Force/1
  Gain3/1 -> Mux1/1
  Gain4/1 -> Mux1/2

== system atrias_on_boom/Mechanical System Layer/L Leg/Mechanical Limits/Shin Min Collision Model ==
  note: Mechanical Limits Model
  phi [rad] : Inport
  vphi [rad/s] : Inport  Port=2
  Contact! : EnablePort  StatesWhenEnabling=reset
  Gain3 : Gain  Gain=sm.k_phi
  Gain4 : Gain  Gain=1/sm.v_phi_max
  Mux1 : Mux  Inputs=2
  Reaction Force : Fcn  Expr="- u(1)  *  (1-u(2)) * (u(2)<1)"
  tau_interaction[Nm] : Outport  OutputWhenDisabled=reset  InitialOutput=0
      settings: AttributesFormatString=initial = '%<InitialOutput>'\nwhen disabled = '%<OutputWhenDisabled>'
  wires:
  Reaction Force/1 -> tau_interaction[Nm]/1
  phi [rad]/1 -> Gain3/1
  vphi [rad/s]/1 -> Gain4/1
  Mux1/1 -> Reaction Force/1
  Gain3/1 -> Mux1/1
  Gain4/1 -> Mux1/2

== system atrias_on_boom/Mechanical System Layer/L Leg/Mechanical Limits/Thigh Max Collision Model ==
  note: Mechanical Limits Model
  phi [rad] : Inport
  vphi [rad/s] : Inport  Port=2
  Contact! : EnablePort  StatesWhenEnabling=reset
  Gain3 : Gain  Gain=sm.k_phi
  Gain4 : Gain  Gain=1/sm.v_phi_max
  Mux1 : Mux  Inputs=2
  Reaction Force : Fcn  Expr="- u(1)  *  (1-u(2)) * (u(2)<1)"
  tau_interaction[Nm] : Outport  OutputWhenDisabled=reset  InitialOutput=0
      settings: AttributesFormatString=initial = '%<InitialOutput>'\nwhen disabled = '%<OutputWhenDisabled>'
  wires:
  Reaction Force/1 -> tau_interaction[Nm]/1
  phi [rad]/1 -> Gain3/1
  vphi [rad/s]/1 -> Gain4/1
  Mux1/1 -> Reaction Force/1
  Gain3/1 -> Mux1/1
  Gain4/1 -> Mux1/2

== system atrias_on_boom/Mechanical System Layer/L Leg/Mechanical Limits/Thigh Min Collision Model ==
  note: Mechanical Limits Model
  phi [rad] : Inport
  vphi [rad/s] : Inport  Port=2
  Contact! : EnablePort  StatesWhenEnabling=reset
  Gain3 : Gain  Gain=sm.k_phi
  Gain4 : Gain  Gain=1/sm.v_phi_max
  Mux1 : Mux  Inputs=2
  Reaction Force : Fcn  Expr="- u(1)  *  (1-u(2)) * (u(2)<1)"
  tau_interaction[Nm] : Outport  OutputWhenDisabled=reset  InitialOutput=0
      settings: AttributesFormatString=initial = '%<InitialOutput>'\nwhen disabled = '%<OutputWhenDisabled>'
  wires:
  Gain4/1 -> Mux1/2
  Gain3/1 -> Mux1/1
  Mux1/1 -> Reaction Force/1
  vphi [rad/s]/1 -> Gain4/1
  phi [rad]/1 -> Gain3/1
  Reaction Force/1 -> tau_interaction[Nm]/1

== system atrias_on_boom/Mechanical System Layer/L Leg/Mechanical Limits/Thigh-Shin Collision Model ==
  note: Mechanical Limits Model
  delta_phi [rad] : Inport
  vphi [rad/s] : Inport  Port=2
  Contact! : EnablePort  StatesWhenEnabling=reset
  Gain3 : Gain  Gain=sm.k_phi
  Gain4 : Gain  Gain=1/sm.v_phi_max
  Mux1 : Mux  Inputs=2
  Reaction Force : Fcn  Expr="- u(1)  *  (1-u(2)) * (u(2)<1)"
  tau_interaction[Nm] : Outport  OutputWhenDisabled=reset  InitialOutput=0
      settings: AttributesFormatString=initial = '%<InitialOutput>'\nwhen disabled = '%<OutputWhenDisabled>'
  wires:
  Gain4/1 -> Mux1/2
  Gain3/1 -> Mux1/1
  Mux1/1 -> Reaction Force/1
  vphi [rad/s]/1 -> Gain4/1
  delta_phi [rad]/1 -> Gain3/1
  Reaction Force/1 -> tau_interaction[Nm]/1

== system atrias_on_boom/Mechanical System Layer/L Leg/Mechanical Limits/Thigh-Shin Collision Model1 ==
  note: Mechanical Limits Model
  delta_phi [rad] : Inport
  vphi [rad/s] : Inport  Port=2
  Contact! : EnablePort  StatesWhenEnabling=reset
  Gain3 : Gain  Gain=sm.k_phi
  Gain4 : Gain  Gain=1/sm.v_phi_max
  Mux1 : Mux  Inputs=2
  Reaction Force : Fcn  Expr="- u(1)  *  (1-u(2)) * (u(2)<1)"
  tau_interaction[Nm] : Outport  OutputWhenDisabled=reset  InitialOutput=0
      settings: AttributesFormatString=initial = '%<InitialOutput>'\nwhen disabled = '%<OutputWhenDisabled>'
  wires:
  Gain4/1 -> Mux1/2
  Gain3/1 -> Mux1/1
  Mux1/1 -> Reaction Force/1
  vphi [rad/s]/1 -> Gain4/1
  delta_phi [rad]/1 -> Gain3/1
  Reaction Force/1 -> tau_interaction[Nm]/1

== system atrias_on_boom/Mechanical System Layer/L Leg/Shin/Frame Data ==
  Kinematic Data : ToWorkspace  VariableName=l_shin_out  SampleTime=sm.output_sample_time
      settings: Save2DSignal=2-D array (concatenate along first dimension)
  Mux : Mux
  PS-Simulink Converter{,1..3} (4 alike) : nesl_utility/PS-Simulink Converter  PhysicalDomain=network_engine_domain  SubClassName=ps_output  LeftPortType=input  RightPortType=output  PseudoPeriodic=off  Frequencies=[]  Unit=1  AffineConversion=off
  Transform Sensor : sm_lib/Frames and Transforms/Transform Sensor  MeasurementFrame=World  SenseAngle=off  SenseAxis=off  SenseAngle1=off  SenseAngle2=off  SenseAngle3=off  SenseQ=on  SenseR=off  SenseOmegaX=off  SenseOmegaY=off  SenseOmegaZ=off  SenseOmega1=off  SenseOmega2=off  SenseOmega3=off  SenseQDot=off  SenseRDot=off  SenseAlphaX=off  SenseAlphaY=off  SenseAlphaZ=off  SenseAlpha1=off  SenseAlpha2=off  SenseAlpha3=off  SenseQDDot=off  SenseRDDot=off  SenseX=on  SenseY=on  SenseZ=on  SenseRad=off  SenseAzim=off  SenseDist=off  SenseInc=off  SenseXDot=off  SenseYDot=off  SenseZDot=off  SenseRadDot=off  SenseAzimDot=off  SenseDistDot=off  SenseIncDot=off  SenseXDDot=off  SenseYDDot=off  SenseZDDot=off  SenseRadDDot=off  SenseAzimDDot=off  SenseDistDDot=off  SenseIncDDot=off
  World Frame : sm_lib/Frames and Transforms/World Frame
  Frame : PMIOPort  Side=Left
  wires:
  PS-Simulink Converter3/1 -> Mux/4
  PS-Simulink Converter2/1 -> Mux/3
  PS-Simulink Converter1/1 -> Mux/2
  PS-Simulink Converter/1 -> Mux/1
  Mux/1 -> Kinematic Data/1
  connections:
  Transform Sensor/LConn1 -- World Frame/RConn1
  Transform Sensor/RConn1 -- Frame/RConn1
  PS-Simulink Converter/LConn1 -- Transform Sensor/RConn2
  PS-Simulink Converter1/LConn1 -- Transform Sensor/RConn3
  PS-Simulink Converter2/LConn1 -- Transform Sensor/RConn4
  PS-Simulink Converter3/LConn1 -- Transform Sensor/RConn5

== system atrias_on_boom/Mechanical System Layer/L Leg/Shin SEA/Motor Controller ==
  Desired Current [A] : Inport
  Measured Current [A] : Inport  Port=2
  Speed [rad/s] : Inport  Port=3
  Ke : Gain  Gain=sm.Kb_leg
  PI Controller : simulink/Continuous/PID Controller  Controller=PI  TimeDomain=Continuous-time  SampleTime=-1  IntegratorMethod=Trapezoidal  FilterMethod=Forward Euler  Form=Parallel  UseFilter=on  ControllerParametersSource=internal  P=0.57  I=0.016  D=0.016  N=10  InitialConditionSource=internal  InitialConditionForIntegrator=0  InitialConditionForFilter=0  ExternalReset=none  ZeroCross=off  LimitOutput=off  UpperSaturationLimit=inf  LowerSaturationLimit=-inf  LinearizeAsGain=on  AntiWindupMode=none  Kb=1  TrackingMode=off  Kt=1  PParamMin=[]  PParamMax=[]  IParamMin=[]  IParamMax=[]  DParamMin=[]  DParamMax=[]  NParamMin=[]  NParamMax=[]  KbParamMin=[]  KbParamMax=[]  KtParamMin=[]  KtParamMax=[]  POutMin=[]  POutMax=[]  IOutMin=[]  IOutMax=[]  DOutMin=[]  DOutMax=[]  NOutMin=[]  NOutMax=[]  KbOutMin=[]  KbOutMax=[]  KtOutMin=[]  KtOutMax=[]  IntegratorOutMin=[]  IntegratorOutMax=[]  FilterOutMin=[]  FilterOutMax=[]  SumOutMin=[]  SumOutMax=[]  SumI1OutMin=[]  SumI1OutMax=[]  SumI2OutMin=[]  SumI2OutMax=[]  SumI3OutMin=[]  SumI3OutMax=[]  SumDOutMin=[]  SumDOutMax=[]  SaturationOutMin=[]  SaturationOutMax=[]  IntegratorContinuousStateAttributes=''  IntegratorStateMustResolveToSignalObject=off  IntegratorRTWStateStorageClass=Auto  FilterContinuousStateAttributes=''  FilterStateMustResolveToSignalObject=off  FilterRTWStateStorageClass=Auto  DifferentiatorICPrevScaledInput=0  DifferentiatorOutMin=[]  DifferentiatorOutMax=[]
  Resistance : Gain  Gain=sm.R_leg
  Sum : Sum  Inputs=|+-
  Sum1 : Sum  Inputs=|++
  Sum2 : Sum  Inputs=+|+
  Voltage [V] : Outport
  wires:
  Sum1/1 -> Voltage [V]/1
  Ke/1 -> Sum2/2
  Resistance/1 -> Sum2/1
  Sum2/1 -> Sum1/2
  Speed [rad/s]/1 -> Ke/1
  PI Controller/1 -> Sum1/1
  Sum/1 -> PI Controller/1
  Measured Current [A]/1 -> Sum/2, Resistance/1
  Desired Current [A]/1 -> Sum/1

== system atrias_on_boom/Mechanical System Layer/L Leg/Shin SEA/Motor Electromagnetism ==
  Voltage [V] : Inport
  Speed [rad/s] : Inport  Port=2
  Add : Sum  Inputs=-+-
  Inductance : Gain  Gain=1/sm.L_leg
  Integrator : Integrator  ZeroCross=off
  Ke : Gain  Gain=sm.Kb_leg
  Resistance : Gain  Gain=sm.R_leg
  Torque Limiter (outside) 1 : Saturate  UpperLimit=sm.max_voltage_leg  LowerLimit=-sm.max_voltage_leg  ZeroCross=off
      settings: AttributesFormatString=Hi: %<UpperLimit>\nLo: %<LowerLimit>
  Torque Limiter (outside) 2 : Saturate  UpperLimit=sm.max_current_leg  LowerLimit=-sm.max_current_leg  ZeroCross=off
      settings: AttributesFormatString=Hi: %<UpperLimit>\nLo: %<LowerLimit>
  Current [A] : Outport
  wires:
  Torque Limiter (outside) 1/1 -> Add/2
  Torque Limiter (outside) 2/1 -> Resistance/1, Current [A]/1
  Voltage [V]/1 -> Torque Limiter (outside) 1/1
  Ke/1 -> Add/3
  Resistance/1 -> Add/1
  Add/1 -> Inductance/1
  Speed [rad/s]/1 -> Ke/1  "d/dt(theta)"
  Inductance/1 -> Integrator/1  "d/dt(I)"
  Integrator/1 -> Torque Limiter (outside) 2/1  "I"
